simulink model "MMMS_v3"  (R2024b)
settings: Solver=VariableStepAuto  StartTime=0.0  StopTime=60  FixedStep=0.001  RelTol=1e-3
InitFcn:
  | %rho_0t=[0.29;0.29;0.29]; %m
  | %V_0t=[-0.001;-0.001;0];%[-0.0005;-0.0005;0];
  | %w_t=[0;0;-0.002];
  | 
  | 
  | %rho_0t=[0.3;0.3;0.2]; %m
  | %V_0t=[-0.001;-0.001;0];%[-0.0005;-0.0005;0];
  | %w_t=[0;0;-0.001];
values from neighbouring files (symbols this model uses):
  Dt = 0.1    [main_EKF.m]
  Fake_Manip_grad = -0.2.*eye(7)    [Initiate_FQ.m]
  g_cm = zeros(4,4,n)    [Initiate_KUKA_inv.m]    (also in Main_MMMS.m; test_KUKA_elements.m)
  g_It00 = [eye(3) rho_It;0 0 0 1]    [main_EKF.m]
  iota0 = eye(6,6)    [Initiate_KUKA_inv.m]    (also in Main_MMMS.m; test_KUKA_elements.m)
  K_d = 10*[1.3*eye(3) zeros(3);zeros(3) 0.8*eye(3)]    [Initiate_FQ.m]    (also in Initiate_KUKA_inv.m = 5*[0.7*eye(3) zeros(3);zeros(3) 0.5*eye(3)]; MMMS_Initiate_FQ.m; Main_MMMS.m = 5*[0.7*eye(3) zeros(3);zeros(3) 0.5*eye(3)]; test_KUKA_elements.m = 50*[0.7*eye(3) zeros(3);zeros(3) 0.5*eye(3)])
  K_i = 5*[0.1*eye(3) zeros(3);zeros(3) 0.01*eye(3)]    [Initiate_FQ.m]    (also in Initiate_KUKA_inv.m = 5*[0.01*eye(3) zeros(3);zeros(3) 0.001*eye(3)]; MMMS_Initiate_FQ.m; Main_MMMS.m = 5*[0.01*eye(3) zeros(3);zeros(3) 0.001*eye(3)]; test_KUKA_elements.m = 50*[0.01*eye(3) zeros(3);zeros(3) 0.001*eye(3)])
  K_p = 100*[0.1 0 0 0 0 0;0 0.1 0 0 0 0; 0 0 0.1 0 0 0; 0 0 0 0.01 0 0 ... (first row only)    [Initiate_FQ.m]    (also in Initiate_KUKA_inv.m = 5*[0.1 0 0 0 0 0;0 0.1 0 0 0 0; 0 0 0.1 0 0 0; 0 0 0 0.01 0 ; MMMS_Initiate_FQ.m; Main_MMMS.m = 5*[0.1 0 0 0 0 0;0 0.1 0 0 0 0; 0 0 0.1 0 0 0; 0 0 0 0.01 0 ; test_KUKA_elements.m = 50*[0.1 0 0 0 0 0;0 0.1 0 0 0 0; 0 0 0.1 0 0 0; 0 0 0 0.01 0)
  K_w = 200*eye(7)    [Initiate_FQ.m]    (also in MMMS_Initiate_FQ.m)
  K_wd = 2*eye(7)    [Initiate_FQ.m]    (also in MMMS_Initiate_FQ.m)
  m = randn(s,total_time_steps,6)*chol(R)    [main_EKF.m]
  M0 = M_temp.M0.data(:,:,1)    [Initiate_FQ.m]    (also in MMMS_Initiate_FQ.m; test_KUKA_elements.m)
  m0 = robot.Bodies{1,n+1}.Mass    [Initiate_KUKA_inv.m]    (also in Main_MMMS.m; test_KUKA_elements.m)
  m0_frak = diag_M(1:6,1:6)    [Initiate_KUKA_inv.m]    (also in Main_MMMS.m; make_uncertain.m = diag_M_unc(1:6,1:6); test_KUKA_elements.m)
  M0m = M_temp.M0m.data(:,:,1)    [Initiate_FQ.m]    (also in MMMS_Initiate_FQ.m; test_KUKA_elements.m)
  m_diag = diag_M(7:end,7:end)    [Initiate_KUKA_inv.m]    (also in Main_MMMS.m; make_uncertain.m = diag_M_unc(7:end,7:end); test_KUKA_elements.m)
  M_t = (((Adjoint(g_It))'\M_t_body)/(Adjoint(g_It)))    [Initiate_FQ.m]    (also in Initiate_KUKA_inv.m = [eye(3)*mt zeros(3); zeros(3) eye(3)*80]; MMMS_Initiate_FQ.m; Main_MMMS.m = [eye(3)*mt zeros(3); zeros(3) eye(3)*80]; test_KUKA_elements.m = [eye(3)*mt zeros(3); zeros(3) eye(3)*80])
  M_t_body = [eye(3)*mt zeros(3); zeros(3) eye(3)*0.416667]    [Initiate_FQ.m]    (also in MMMS_Initiate_FQ.m)
  mm = zeros(1,n)    [Initiate_KUKA_inv.m]    (also in Main_MMMS.m; test_KUKA_elements.m)
  mu = P0    [Initiate_FQ.m]    (also in Initiate_KUKA_inv.m = zeros(6,1); MMMS_Initiate_FQ.m; Main_MMMS.m = zeros(6,1); make_uncertain.m = P0_unc)
  mu_t = inv((Adjoint(g_It))')*M_t_body*[V_It;w_t]    [Initiate_FQ.m]    (also in Initiate_KUKA_inv.m = M_t*[V_0t;w_t]; MMMS_Initiate_FQ.m; Main_MMMS.m = M_t*[V_0t;w_t]; make_uncertain.m = inv((Adjoint(g_It))')*M_t_body_unc*[V_It;w_t])
  noise_st = 0.000005    (= 5e-06)    [main_EKF.m]
  q_dot_m = [0;0;0;0;0;0;0]    [Initiate_FQ.m]    (also in Initiate_KUKA_inv.m; MMMS_Initiate_FQ.m; Main_MMMS.m; test_KUKA_elements.m = [0])
  q_m = [0.2;1.2;0.3;2.5;0.5;1.5;0.6]    [Initiate_FQ.m]    (also in Initiate_KUKA_inv.m = [0;0;0;0;0;0;0]; MMMS_Initiate_FQ.m = [0.2;0.2;0.3;0.5;0.5;0.5;0.6]; Main_MMMS.m = [0;0;0;0;0;0;0]; test_KUKA_elements.m = [0.2;1.2;0.3;1.8;0.5;1.3;0.6])
  rho_It = [0;0;1.7]    [Initiate_FQ.m]    (also in MMMS_Initiate_FQ.m)
  s = RandStream.create('mrg32k3a','NumStreams',1)    [main_EKF.m]
  sc_size = 1    [Initiate_KUKA_inv.m]    (also in Main_MMMS.m; test_KUKA_elements.m)
  V_It = [0.0005;0.0005;0]    [Initiate_FQ.m]    (also in MMMS_Initiate_FQ.m = [0.001;0.001;0])
  Xi_m_matrix = zeros(6*n,n)    [Initiate_KUKA_inv.m]    (also in Main_MMMS.m)
undefined symbols (not defined in the file or in its folder): g_cm0, I0, Im, Mm, X, Xi_m, Y, Z
libraries: nesl_utility x314, sm_lib x231, robotcorelib x30, simulink x12
(part 2 of 13)

== system MMMS_v3/Feedback Transformation1 ==
  note: Feedback Transformation
  g_I0 : Inport
  q_m : Inport  Port=2
  U_c2 : Inport  Port=3
  f_N : Inport  Port=4
  CBF_m : Inport  Port=5
  Add1 : Sum  Inputs=+++++++
  Bus Selector1 : BusSelector  OutputSignals=signal2
  Constant1 : Constant  Value=mu
  Constant4 : Constant  Value=mu_t
  Gain10 : Gain
  Gain5 : Gain  Gain=0
  Gain7 : Gain  Gain=0
  Gain8 : Gain
  Gain9 : Gain  Gain=0
  Inverse Dynamics1 : Subsystem
  Matrix Multiply{1..3,8} (4 alike) : Product  Multiplication=Matrix(*)
  f_m : Outport
  tag scope: fm2=global
  wires:
  q_m/1 -> Inverse Dynamics1/2("q_m "), Bus Selector1/1
  g_I0/1 -> Inverse Dynamics1/1(g_I0)
  Gain8/1 -> Add1/5
  Inverse Dynamics1/3(F_t) -> Matrix Multiply8/1
  Inverse Dynamics1/4(F_m) -> Matrix Multiply1/1
  Gain9/1 -> Add1/4
  Constant4/1 -> Matrix Multiply8/2  "mu_t"
  Add1/1 -> [fm2], f_m/1  "f_m"
  Bus Selector1/1 -> Matrix Multiply1/2  "<signal2>"
  f_N/1 -> Gain10/1
  Gain5/1 -> Add1/1
  Matrix Multiply3/1 -> Gain9/1
  Matrix Multiply8/1 -> Gain8/1
  Inverse Dynamics1/5(N) -> Gain5/1
  U_c2/1 -> Matrix Multiply2/2
  Constant1/1 -> Matrix Multiply3/2  "mu"
  Inverse Dynamics1/1(F_U) -> Matrix Multiply2/1
  Gain10/1 -> Add1/6
  Matrix Multiply1/1 -> Gain7/1
  Gain7/1 -> Add1/2
  Inverse Dynamics1/2(F_mu) -> Matrix Multiply3/1
  CBF_m/1 -> Add1/7
  Matrix Multiply2/1 -> Add1/3  "f_m"

== system MMMS_v3/Feedback Transformation2 ==
  note: Feedback Transformation
  g_I0 : Inport
  q_m : Inport  Port=2
  U_c2 : Inport  Port=3
  f_N : Inport  Port=4
  Add1 : Sum  Inputs=++++++
  Bus Selector1 : BusSelector  OutputSignals=signal2
  Constant1 : Constant  Value=mu
  Constant4 : Constant  Value=mu_t
  Gain10 : Gain
  Gain5 : Gain  Gain=0
  Gain7 : Gain  Gain=0
  Gain8 : Gain
  Gain9 : Gain  Gain=0
  Inverse Dynamics1 : Subsystem
  Matrix Multiply{1..3,8} (4 alike) : Product  Multiplication=Matrix(*)
  f_m : Outport
  tag scope: fm3=global
  wires:
  Inverse Dynamics1/2(F_mu) -> Matrix Multiply3/1
  Gain7/1 -> Add1/2
  Matrix Multiply1/1 -> Gain7/1
  Gain10/1 -> Add1/6
  Inverse Dynamics1/1(F_U) -> Matrix Multiply2/1
  Constant1/1 -> Matrix Multiply3/2  "mu"
  U_c2/1 -> Matrix Multiply2/2
  Inverse Dynamics1/5(N) -> Gain5/1
  Matrix Multiply8/1 -> Gain8/1
  Matrix Multiply3/1 -> Gain9/1
  Gain5/1 -> Add1/1
  f_N/1 -> Gain10/1
  Matrix Multiply2/1 -> Add1/3  "f_m"
  Bus Selector1/1 -> Matrix Multiply1/2  "<signal2>"
  Add1/1 -> [fm3], f_m/1  "f_m"
  Constant4/1 -> Matrix Multiply8/2  "mu_t"
  Gain9/1 -> Add1/4
  Inverse Dynamics1/4(F_m) -> Matrix Multiply1/1
  Inverse Dynamics1/3(F_t) -> Matrix Multiply8/1
  Gain8/1 -> Add1/5
  g_I0/1 -> Inverse Dynamics1/1(g_I0)
  q_m/1 -> Bus Selector1/1, Inverse Dynamics1/2("q_m ")

== system MMMS_v3/Inverse Dynamics ==
  note: f_m
  g_I0 : Inport
  "q_m " : Inport  Port=2
  A_dot : MATLAB Function  TreatAsAtomicUnit=on
  Bus Selector : BusSelector  OutputSignals=M0,Mm
  Bus Selector2 : BusSelector  OutputSignals=signal1,signal2
  C_hat : Subsystem  Commented=on
  C_hat1 : Subsystem
  Inverse Dynamics : Subsystem
  M0_dot : MATLAB Function  TreatAsAtomicUnit=on
  N_hat : Subsystem  Commented=on
  N_hat1 : Subsystem
  Scope : Scope
  F_U : Outport
  F_mu : Outport  Port=2
  F_t : Outport  Port=3
  F_m : Outport  Port=4
  N : Outport  Port=5
  wires:
  [P] -> N_hat1/5(P)
  [Mass_Matrix] -> Bus Selector/1
  Bus Selector/1 -> N_hat1/6(M0), Inverse Dynamics/2(<M0>)  "<M0>"
  g_I0/1 -> N_hat1/1(g_I0), Inverse Dynamics/1(g_I0)
  Inverse Dynamics/1(F_U) -> F_U/1
  Inverse Dynamics/2(F_mu) -> F_mu/1
  Inverse Dynamics/3(F_t) -> F_t/1
  Inverse Dynamics/4(F_m) -> F_m/1
  Bus Selector/2 -> Inverse Dynamics/3(Mm)  "<Mm>"
  Bus Selector2/1 -> N_hat1/2(q_m), C_hat1/1(q_m)  "<signal1>"
  Bus Selector2/2 -> A_dot/2(q_m_dot), M0_dot/2(q_m_dot), N_hat1/3(q_dot_m), C_hat1/2(q_dot_m)  "<signal2>"
  C_hat1/1(M0_partial) -> M0_dot/1(M0_partial)
  C_hat1/2(Out1) -> A_dot/1(A_partial)
  C_hat1/3(C_hat1) -> Inverse Dynamics/6(C_hat)
  M0_dot/1(M0_dot) -> Inverse Dynamics/4(M0_dot)
  A_dot/1(A_dot) -> Inverse Dynamics/5(A_dot)
  "q_m "/1 -> Bus Selector2/1
  [A_connection] -> N_hat1/4(A)
  N_hat1/1(N_hat1) -> N/1, Scope/1

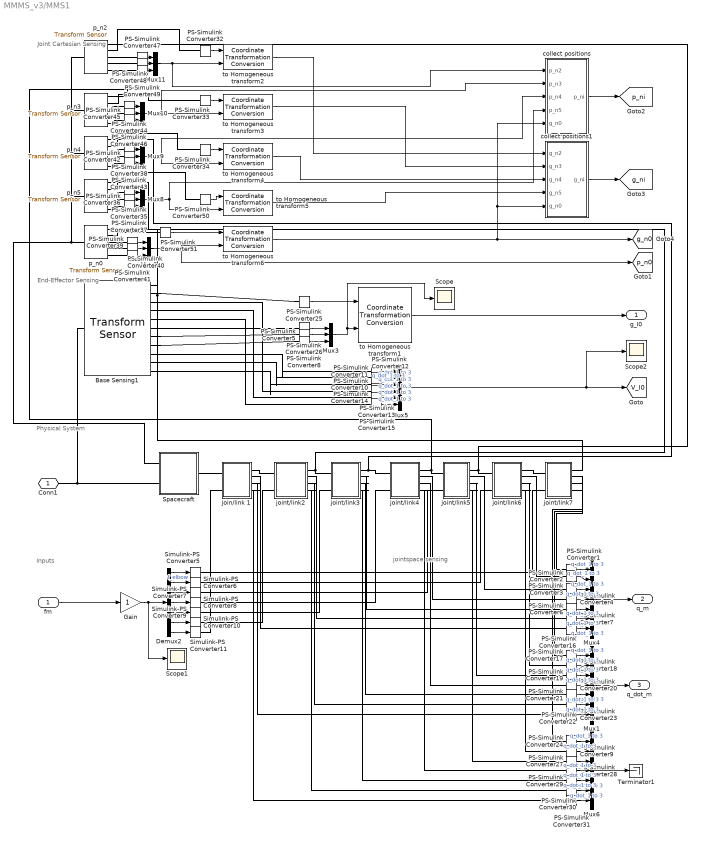
== system MMMS_v3/MMS1 ==
  note: Physical System
  note: jointspace sensing
  note: Inputs
  note: End-Effector Sensing
  note: Joint Cartesian Sensing
  fm : Inport
  Base Sensing1 : sm_lib/Frames and Transforms/Transform Sensor  MeasurementFrame=NonRotatingBase  RotationSequence=XYZ  SenseAngle=off  SenseAxis=off  SenseQ=off  SenseR=on  SenseRotationSequence=off  SenseOmegaX=on  SenseOmegaY=on  SenseOmegaZ=on  SenseOmega=off  SenseQDot=off  SenseRDot=off  SenseRotationSequenceDot=off  SenseAlphaX=off  SenseAlphaY=off  SenseAlphaZ=off  SenseAlpha=off  SenseQDDot=off  SenseRDDot=off  SenseX=on  SenseY=on  SenseZ=on  SenseXYZ=off  SenseRad=off  SenseAzim=off  SenseDist=off  SenseInc=off  SenseXDot=on  SenseYDot=on  SenseZDot=on  SenseXYZDot=off  SenseRadDot=off  SenseAzimDot=off  SenseDistDot=off  SenseIncDot=off  SenseXDDot=off  SenseYDDot=off  SenseZDDot=off  SenseXYZDDot=off  SenseRadDDot=off  SenseAzimDDot=off  SenseDistDDot=off  SenseIncDDot=off
  Demux2 : Demux  Outputs=7
  Gain : Gain
  Mux1 : Mux  Inputs=7
  Mux{2..3,8..11} (6 alike) : Mux  Inputs=3
  Mux4 : Mux  Inputs=7
  Mux5 : Mux  Inputs=6
  Mux6 : Mux  Inputs=7
  PS-Simulink Converter{1..51} (51 alike) : nesl_utility/PS-Simulink Converter  PhysicalDomain=network_engine_domain  SubClassName=ps_output  LeftPortType=input  RightPortType=output  PseudoPeriodic=off  Frequencies=[]  VectorFormat=1-D array  Unit=inherit  AffineConversion=off
  Scope : Scope
  Scope1 : Scope
  Scope2 : Scope
  Simulink-PS Converter{5..11} (7 alike) : nesl_utility/Simulink-PS Converter  PhysicalDomain=network_engine_domain  SubClassName=ps_input  LeftPortType=input  RightPortType=output  PseudoPeriodic=off  Frequencies=[]  NoiseDistribution=none  NoiseParameters=[]  Unit=1  AffineConversion=off  FilteringAndDerivatives=provide  SimscapeFilterOrder=1  InputFilterTimeConstant=0.001  UdotUserProvided=0
  Spacecraft : Subsystem
  Terminator1 : Terminator
  collect positions : MATLAB Function  TreatAsAtomicUnit=on
  collect positions1 : MATLAB Function  TreatAsAtomicUnit=on
  join/link 1 : Subsystem
  joint/link2 : Subsystem
  joint/link3 : Subsystem
  joint/link4 : Subsystem
  joint/link5 : Subsystem
  joint/link6 : Subsystem
  joint/link7 : Subsystem
  p_n{0,2..5} (5 alike) : sm_lib/Frames and Transforms/Transform Sensor  MeasurementFrame=Base  RotationSequence=XYZ  SenseAngle=off  SenseAxis=off  SenseQ=off  SenseR=on  SenseRotationSequence=off  SenseOmegaX=off  SenseOmegaY=off  SenseOmegaZ=off  SenseOmega=off  SenseQDot=off  SenseRDot=off  SenseRotationSequenceDot=off  SenseAlphaX=off  SenseAlphaY=off  SenseAlphaZ=off  SenseAlpha=off  SenseQDDot=off  SenseRDDot=off  SenseX=on  SenseY=on  SenseZ=on  SenseXYZ=off  SenseRad=off  SenseAzim=off  SenseDist=off  SenseInc=off  SenseXDot=off  SenseYDot=off  SenseZDot=off  SenseXYZDot=off  SenseRadDot=off  SenseAzimDot=off  SenseDistDot=off  SenseIncDot=off  SenseXDDot=off  SenseYDDot=off  SenseZDDot=off  SenseXYZDDot=off  SenseRadDDot=off  SenseAzimDDot=off  SenseDistDDot=off  SenseIncDDot=off
  to Homogeneous transform{1..6} (6 alike) : robotcorelib/Coordinate Transformation Conversion  InputRepresentation=Rotation Matrix  InputEulerSequence=ZYX  ShowTrVecInputPort=on  OutputRepresentation=Homogeneous Transformation  OutputEulerSequence=ZYX  ShowTrVecOutputPort=on  SimulateUsing=Code generation
  Conn1 : PMIOPort  Side=Left
  g_I0 : Outport
  q_m : Outport  Port=2
  q_dot_m : Outport  Port=3
  tag scope: V_I0=global, g_n0=global, g_ni=global, p_n0=global, p_ni=global
  wires:
  Demux2/1 -> Simulink-PS Converter5/1
  Demux2/3 -> Simulink-PS Converter7/1
  PS-Simulink Converter15/1 -> Mux5/6  "q_dot_1 to 3"
  PS-Simulink Converter10/1 -> Mux5/3  "q_dot_1 to 3"
  fm/1 -> Gain/1
  PS-Simulink Converter25/1 -> to Homogeneous transform1/1
  Gain/1 -> Scope1/1, Demux2/1
  PS-Simulink Converter8/1 -> Mux3/3
  Mux3/1 -> Scope/1, to Homogeneous transform1/2
  PS-Simulink Converter12/1 -> Mux5/2  "q_dot_1 to 3"
  to Homogeneous transform1/1 -> g_I0/1
  PS-Simulink Converter13/1 -> Mux5/4  "q_dot_1 to 3"
  PS-Simulink Converter26/1 -> Mux3/1
  Demux2/7 -> Simulink-PS Converter11/1
  PS-Simulink Converter14/1 -> Mux5/5  "q_dot_1 to 3"
  Demux2/4 -> Simulink-PS Converter8/1
  PS-Simulink Converter11/1 -> Mux5/1  "q_dot_1 to 3"
  PS-Simulink Converter5/1 -> Mux3/2
  Demux2/6 -> Simulink-PS Converter10/1
  Demux2/2 -> Simulink-PS Converter6/1  "f_elbow"
  Demux2/5 -> Simulink-PS Converter9/1
  PS-Simulink Converter27/1 -> Mux6/3  "q_dot_1 to 3"
  PS-Simulink Converter1/1 -> Mux4/1  "q_dot_1 to 3"
  PS-Simulink Converter6/1 -> Mux4/5  "q_dot_1 to 3"
  PS-Simulink Converter30/1 -> Mux6/6  "q_dot_1 to 3"
  PS-Simulink Converter3/1 -> Mux4/3  "q_dot_1 to 3"
  PS-Simulink Converter18/1 -> Mux1/2  "q_dot_1 to 3"
  PS-Simulink Converter31/1 -> Mux6/7  "q_dot_1 to 3"
  PS-Simulink Converter9/1 -> Mux6/2  "q_dot_1 to 3"
  PS-Simulink Converter7/1 -> Mux4/6  "q_dot_1 to 3"
  PS-Simulink Converter2/1 -> Mux4/2  "q_dot_1 to 3"
  PS-Simulink Converter4/1 -> Mux4/4  "q_dot_1 to 3"
  PS-Simulink Converter21/1 -> Mux1/5  "q_dot_1 to 3"
  PS-Simulink Converter23/1 -> Mux1/7  "q_dot_1 to 3"
  PS-Simulink Converter16/1 -> Mux4/7  "q_dot_1 to 3"
  PS-Simulink Converter28/1 -> Mux6/4  "q_dot_1 to 3"
  Mux4/1 -> q_m/1
  Mux1/1 -> q_dot_m/1
  PS-Simulink Converter24/1 -> Mux6/1  "q_dot_1 to 3"
  Mux6/1 -> Terminator1/1
  PS-Simulink Converter20/1 -> Mux1/4  "q_dot_1 to 3"
  PS-Simulink Converter29/1 -> Mux6/5  "q_dot_1 to 3"
  PS-Simulink Converter22/1 -> Mux1/6  "q_dot_1 to 3"
  PS-Simulink Converter17/1 -> Mux1/1  "q_dot_1 to 3"
  PS-Simulink Converter19/1 -> Mux1/3  "q_dot_1 to 3"
  Mux5/1 -> [V_I0], Scope2/1
  Mux2/1 -> to Homogeneous transform6/2, [p_n0]
  PS-Simulink Converter39/1 -> Mux2/1
  PS-Simulink Converter40/1 -> Mux2/2
  PS-Simulink Converter41/1 -> Mux2/3
  PS-Simulink Converter36/1 -> Mux8/2
  PS-Simulink Converter35/1 -> Mux8/1
  PS-Simulink Converter37/1 -> Mux8/3
  PS-Simulink Converter42/1 -> Mux9/2
  PS-Simulink Converter38/1 -> Mux9/1
  PS-Simulink Converter43/1 -> Mux9/3
  PS-Simulink Converter45/1 -> Mux10/2
  PS-Simulink Converter44/1 -> Mux10/1
  PS-Simulink Converter46/1 -> Mux10/3
  Mux11/1 -> to Homogeneous transform2/2, collect positions/1(p_n2)
  PS-Simulink Converter48/1 -> Mux11/2
  PS-Simulink Converter47/1 -> Mux11/1
  PS-Simulink Converter49/1 -> Mux11/3
  collect positions/1(p_ni) -> [p_ni]
  PS-Simulink Converter32/1 -> to Homogeneous transform2/1
  PS-Simulink Converter33/1 -> to Homogeneous transform3/1
  Mux10/1 -> to Homogeneous transform3/2, collect positions/2(p_n3)
  Mux9/1 -> to Homogeneous transform4/2, collect positions/3(p_n4)
  PS-Simulink Converter34/1 -> to Homogeneous transform4/1
  PS-Simulink Converter50/1 -> to Homogeneous transform5/1
  Mux8/1 -> to Homogeneous transform5/2, collect positions/4(p_n5)
  collect positions1/1(g_ni) -> [g_ni]
  PS-Simulink Converter51/1 -> to Homogeneous transform6/1
  to Homogeneous transform6/1 -> collect positions/5(g_n0), collect positions1/5(g_n0), [g_n0]
  to Homogeneous transform2/1 -> collect positions1/1(g_n2)
  to Homogeneous transform3/1 -> collect positions1/2(g_n3)
  to Homogeneous transform4/1 -> collect positions1/3(g_n4)
  to Homogeneous transform5/1 -> collect positions1/4(g_n5)
  connections:
  Spacecraft/LConn2 -- Conn1/RConn1 -- Base Sensing1/LConn1
  p_n0/RConn1 -- joint/link7/RConn1 -- Base Sensing1/RConn1
  joint/link4/LConn1 -- p_n4/RConn1 -- joint/link3/RConn1
  Base Sensing1/RConn10 -- PS-Simulink Converter12/LConn1
  Simulink-PS Converter9/RConn1 -- joint/link3/LConn2
  Simulink-PS Converter8/RConn1 -- joint/link4/LConn2
  Base Sensing1/RConn2 -- PS-Simulink Converter25/LConn1
  joint/link5/LConn1 -- joint/link4/RConn1 -- p_n3/RConn1
  Base Sensing1/RConn5 -- PS-Simulink Converter15/LConn1
  Base Sensing1/RConn7 -- PS-Simulink Converter5/LConn1
  joint/link6/LConn1 -- joint/link5/RConn1 -- p_n2/RConn1
  Base Sensing1/RConn11 -- PS-Simulink Converter10/LConn1
  Base Sensing1/RConn3 -- PS-Simulink Converter13/LConn1
  Simulink-PS Converter5/RConn1 -- joint/link7/LConn2
  Base Sensing1/RConn4 -- PS-Simulink Converter14/LConn1
  Base Sensing1/RConn9 -- PS-Simulink Converter11/LConn1
  Base Sensing1/RConn8 -- PS-Simulink Converter8/LConn1
  Base Sensing1/RConn6 -- PS-Simulink Converter26/LConn1
  Simulink-PS Converter7/RConn1 -- joint/link5/LConn2
  joint/link6/RConn3 -- PS-Simulink Converter18/LConn1
  joint/link6/RConn4 -- PS-Simulink Converter9/LConn1
  joint/link5/RConn2 -- PS-Simulink Converter3/LConn1
  joint/link5/RConn3 -- PS-Simulink Converter19/LConn1
  joint/link5/RConn4 -- PS-Simulink Converter27/LConn1
  joint/link4/RConn2 -- PS-Simulink Converter4/LConn1
  joint/link4/RConn3 -- PS-Simulink Converter20/LConn1
  joint/link4/RConn4 -- PS-Simulink Converter28/LConn1
  joint/link3/RConn2 -- PS-Simulink Converter6/LConn1
  joint/link3/RConn3 -- PS-Simulink Converter21/LConn1
  joint/link3/RConn4 -- PS-Simulink Converter29/LConn1
  joint/link6/RConn1 -- joint/link7/LConn1
  joint/link6/RConn2 -- PS-Simulink Converter2/LConn1
  joint/link6/LConn2 -- Simulink-PS Converter6/RConn1
  joint/link7/RConn2 -- PS-Simulink Converter1/LConn1
  joint/link7/RConn3 -- PS-Simulink Converter17/LConn1
  joint/link7/RConn4 -- PS-Simulink Converter24/LConn1
  join/link 1/LConn2 -- Simulink-PS Converter11/RConn1
  join/link 1/LConn1 -- Spacecraft/RConn1
  join/link 1/RConn1 -- joint/link2/LConn1
  Simulink-PS Converter10/RConn1 -- joint/link2/LConn2
  joint/link3/LConn1 -- p_n5/RConn1 -- joint/link2/RConn1
  join/link 1/RConn2 -- PS-Simulink Converter16/LConn1
  PS-Simulink Converter7/LConn1 -- joint/link2/RConn2
  joint/link2/RConn4 -- PS-Simulink Converter30/LConn1
  join/link 1/RConn4 -- PS-Simulink Converter31/LConn1
  joint/link2/RConn3 -- PS-Simulink Converter22/LConn1
  join/link 1/RConn3 -- PS-Simulink Converter23/LConn1
  PS-Simulink Converter41/LConn1 -- p_n0/RConn5
  p_n0/RConn4 -- PS-Simulink Converter40/LConn1
  Spacecraft/LConn1 -- p_n2/LConn1 -- p_n3/LConn1 -- p_n4/LConn1 -- p_n5/LConn1 -- p_n0/LConn1
  p_n0/RConn3 -- PS-Simulink Converter39/LConn1
  PS-Simulink Converter37/LConn1 -- p_n5/RConn5
  p_n5/RConn3 -- PS-Simulink Converter35/LConn1
  p_n5/RConn4 -- PS-Simulink Converter36/LConn1
  PS-Simulink Converter43/LConn1 -- p_n4/RConn5
  p_n4/RConn3 -- PS-Simulink Converter38/LConn1
  p_n4/RConn4 -- PS-Simulink Converter42/LConn1
  PS-Simulink Converter46/LConn1 -- p_n3/RConn5
  p_n3/RConn3 -- PS-Simulink Converter44/LConn1
  p_n3/RConn4 -- PS-Simulink Converter45/LConn1
  PS-Simulink Converter49/LConn1 -- p_n2/RConn5
  p_n2/RConn3 -- PS-Simulink Converter47/LConn1
  p_n2/RConn4 -- PS-Simulink Converter48/LConn1
  PS-Simulink Converter32/LConn1 -- p_n2/RConn2
  p_n3/RConn2 -- PS-Simulink Converter33/LConn1
  p_n4/RConn2 -- PS-Simulink Converter34/LConn1
  p_n5/RConn2 -- PS-Simulink Converter50/LConn1
  p_n0/RConn2 -- PS-Simulink Converter51/LConn1

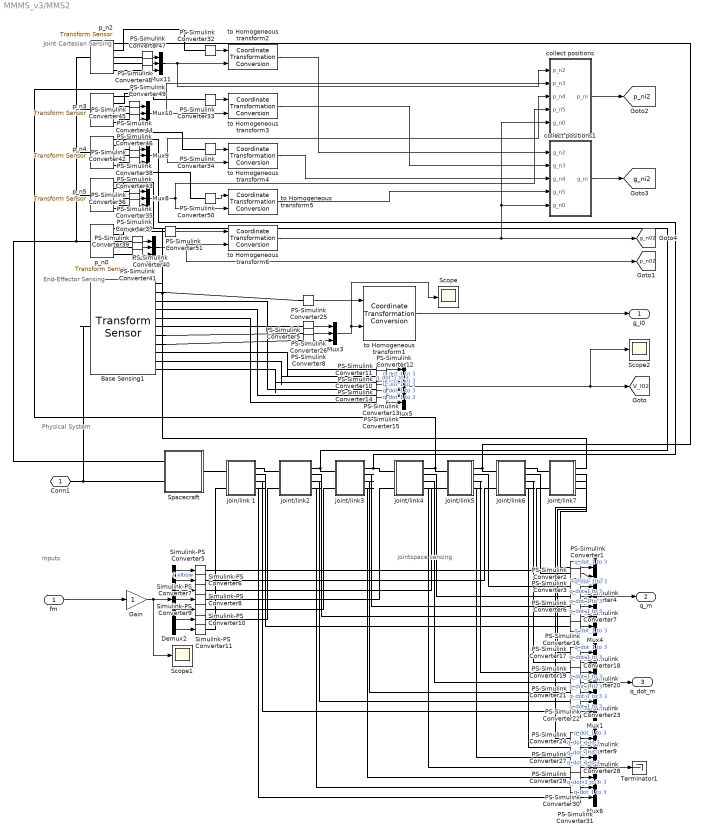
== system MMMS_v3/MMS2 ==
  note: Joint Cartesian Sensing
  note: End-Effector Sensing
  note: Inputs
  note: jointspace sensing
  note: Physical System
  fm : Inport
  Base Sensing1 : sm_lib/Frames and Transforms/Transform Sensor  MeasurementFrame=NonRotatingBase  RotationSequence=XYZ  SenseAngle=off  SenseAxis=off  SenseQ=off  SenseR=on  SenseRotationSequence=off  SenseOmegaX=on  SenseOmegaY=on  SenseOmegaZ=on  SenseOmega=off  SenseQDot=off  SenseRDot=off  SenseRotationSequenceDot=off  SenseAlphaX=off  SenseAlphaY=off  SenseAlphaZ=off  SenseAlpha=off  SenseQDDot=off  SenseRDDot=off  SenseX=on  SenseY=on  SenseZ=on  SenseXYZ=off  SenseRad=off  SenseAzim=off  SenseDist=off  SenseInc=off  SenseXDot=on  SenseYDot=on  SenseZDot=on  SenseXYZDot=off  SenseRadDot=off  SenseAzimDot=off  SenseDistDot=off  SenseIncDot=off  SenseXDDot=off  SenseYDDot=off  SenseZDDot=off  SenseXYZDDot=off  SenseRadDDot=off  SenseAzimDDot=off  SenseDistDDot=off  SenseIncDDot=off
  Demux2 : Demux  Outputs=7
  Gain : Gain
  Mux1 : Mux  Inputs=7
  Mux{2..3,8..11} (6 alike) : Mux  Inputs=3
  Mux4 : Mux  Inputs=7
  Mux5 : Mux  Inputs=6
  Mux6 : Mux  Inputs=7
  PS-Simulink Converter{1..51} (51 alike) : nesl_utility/PS-Simulink Converter  PhysicalDomain=network_engine_domain  SubClassName=ps_output  LeftPortType=input  RightPortType=output  PseudoPeriodic=off  Frequencies=[]  VectorFormat=1-D array  Unit=inherit  AffineConversion=off
  Scope : Scope
  Scope1 : Scope
  Scope2 : Scope
  Simulink-PS Converter{5..11} (7 alike) : nesl_utility/Simulink-PS Converter  PhysicalDomain=network_engine_domain  SubClassName=ps_input  LeftPortType=input  RightPortType=output  PseudoPeriodic=off  Frequencies=[]  NoiseDistribution=none  NoiseParameters=[]  Unit=1  AffineConversion=off  FilteringAndDerivatives=provide  SimscapeFilterOrder=1  InputFilterTimeConstant=0.001  UdotUserProvided=0
  Spacecraft : Subsystem
  Terminator1 : Terminator
  collect positions : MATLAB Function  TreatAsAtomicUnit=on
  collect positions1 : MATLAB Function  TreatAsAtomicUnit=on
  join/link 1 : Subsystem
  joint/link2 : Subsystem
  joint/link3 : Subsystem
  joint/link4 : Subsystem
  joint/link5 : Subsystem
  joint/link6 : Subsystem
  joint/link7 : Subsystem
  p_n{0,2..5} (5 alike) : sm_lib/Frames and Transforms/Transform Sensor  MeasurementFrame=Base  RotationSequence=XYZ  SenseAngle=off  SenseAxis=off  SenseQ=off  SenseR=on  SenseRotationSequence=off  SenseOmegaX=off  SenseOmegaY=off  SenseOmegaZ=off  SenseOmega=off  SenseQDot=off  SenseRDot=off  SenseRotationSequenceDot=off  SenseAlphaX=off  SenseAlphaY=off  SenseAlphaZ=off  SenseAlpha=off  SenseQDDot=off  SenseRDDot=off  SenseX=on  SenseY=on  SenseZ=on  SenseXYZ=off  SenseRad=off  SenseAzim=off  SenseDist=off  SenseInc=off  SenseXDot=off  SenseYDot=off  SenseZDot=off  SenseXYZDot=off  SenseRadDot=off  SenseAzimDot=off  SenseDistDot=off  SenseIncDot=off  SenseXDDot=off  SenseYDDot=off  SenseZDDot=off  SenseXYZDDot=off  SenseRadDDot=off  SenseAzimDDot=off  SenseDistDDot=off  SenseIncDDot=off
  to Homogeneous transform{1..6} (6 alike) : robotcorelib/Coordinate Transformation Conversion  InputRepresentation=Rotation Matrix  InputEulerSequence=ZYX  ShowTrVecInputPort=on  OutputRepresentation=Homogeneous Transformation  OutputEulerSequence=ZYX  ShowTrVecOutputPort=on  SimulateUsing=Code generation
  Conn1 : PMIOPort  Side=Left
  g_I0 : Outport
  q_m : Outport  Port=2
  q_dot_m : Outport  Port=3
  tag scope: V_I02=global, g_n02=global, g_ni2=global, p_n02=global, p_ni2=global
  wires:
  to Homogeneous transform5/1 -> collect positions1/4(g_n5)
  to Homogeneous transform4/1 -> collect positions1/3(g_n4)
  to Homogeneous transform3/1 -> collect positions1/2(g_n3)
  to Homogeneous transform2/1 -> collect positions1/1(g_n2)
  to Homogeneous transform6/1 -> [g_n02], collect positions1/5(g_n0), collect positions/5(g_n0)
  PS-Simulink Converter51/1 -> to Homogeneous transform6/1
  collect positions1/1(g_ni) -> [g_ni2]
  Mux8/1 -> collect positions/4(p_n5), to Homogeneous transform5/2
  PS-Simulink Converter50/1 -> to Homogeneous transform5/1
  PS-Simulink Converter34/1 -> to Homogeneous transform4/1
  Mux9/1 -> collect positions/3(p_n4), to Homogeneous transform4/2
  Mux10/1 -> collect positions/2(p_n3), to Homogeneous transform3/2
  PS-Simulink Converter33/1 -> to Homogeneous transform3/1
  PS-Simulink Converter32/1 -> to Homogeneous transform2/1
  collect positions/1(p_ni) -> [p_ni2]
  PS-Simulink Converter49/1 -> Mux11/3
  PS-Simulink Converter47/1 -> Mux11/1
  PS-Simulink Converter48/1 -> Mux11/2
  Mux11/1 -> collect positions/1(p_n2), to Homogeneous transform2/2
  PS-Simulink Converter46/1 -> Mux10/3
  PS-Simulink Converter44/1 -> Mux10/1
  PS-Simulink Converter45/1 -> Mux10/2
  PS-Simulink Converter43/1 -> Mux9/3
  PS-Simulink Converter38/1 -> Mux9/1
  PS-Simulink Converter42/1 -> Mux9/2
  PS-Simulink Converter37/1 -> Mux8/3
  PS-Simulink Converter35/1 -> Mux8/1
  PS-Simulink Converter36/1 -> Mux8/2
  PS-Simulink Converter41/1 -> Mux2/3
  PS-Simulink Converter40/1 -> Mux2/2
  PS-Simulink Converter39/1 -> Mux2/1
  Mux2/1 -> [p_n02], to Homogeneous transform6/2
  Mux5/1 -> Scope2/1, [V_I02]
  PS-Simulink Converter19/1 -> Mux1/3  "q_dot_1 to 3"
  PS-Simulink Converter17/1 -> Mux1/1  "q_dot_1 to 3"
  PS-Simulink Converter22/1 -> Mux1/6  "q_dot_1 to 3"
  PS-Simulink Converter29/1 -> Mux6/5  "q_dot_1 to 3"
  PS-Simulink Converter20/1 -> Mux1/4  "q_dot_1 to 3"
  Mux6/1 -> Terminator1/1
  PS-Simulink Converter24/1 -> Mux6/1  "q_dot_1 to 3"
  Mux1/1 -> q_dot_m/1
  Mux4/1 -> q_m/1
  PS-Simulink Converter28/1 -> Mux6/4  "q_dot_1 to 3"
  PS-Simulink Converter16/1 -> Mux4/7  "q_dot_1 to 3"
  PS-Simulink Converter23/1 -> Mux1/7  "q_dot_1 to 3"
  PS-Simulink Converter21/1 -> Mux1/5  "q_dot_1 to 3"
  PS-Simulink Converter4/1 -> Mux4/4  "q_dot_1 to 3"
  PS-Simulink Converter2/1 -> Mux4/2  "q_dot_1 to 3"
  PS-Simulink Converter7/1 -> Mux4/6  "q_dot_1 to 3"
  PS-Simulink Converter9/1 -> Mux6/2  "q_dot_1 to 3"
  PS-Simulink Converter31/1 -> Mux6/7  "q_dot_1 to 3"
  PS-Simulink Converter18/1 -> Mux1/2  "q_dot_1 to 3"
  PS-Simulink Converter3/1 -> Mux4/3  "q_dot_1 to 3"
  PS-Simulink Converter30/1 -> Mux6/6  "q_dot_1 to 3"
  PS-Simulink Converter6/1 -> Mux4/5  "q_dot_1 to 3"
  PS-Simulink Converter1/1 -> Mux4/1  "q_dot_1 to 3"
  PS-Simulink Converter27/1 -> Mux6/3  "q_dot_1 to 3"
  Demux2/5 -> Simulink-PS Converter9/1
  Demux2/2 -> Simulink-PS Converter6/1  "f_elbow"
  Demux2/6 -> Simulink-PS Converter10/1
  PS-Simulink Converter5/1 -> Mux3/2
  PS-Simulink Converter11/1 -> Mux5/1  "q_dot_1 to 3"
  Demux2/4 -> Simulink-PS Converter8/1
  PS-Simulink Converter14/1 -> Mux5/5  "q_dot_1 to 3"
  Demux2/7 -> Simulink-PS Converter11/1
  PS-Simulink Converter26/1 -> Mux3/1
  PS-Simulink Converter13/1 -> Mux5/4  "q_dot_1 to 3"
  to Homogeneous transform1/1 -> g_I0/1
  PS-Simulink Converter12/1 -> Mux5/2  "q_dot_1 to 3"
  Mux3/1 -> to Homogeneous transform1/2, Scope/1
  PS-Simulink Converter8/1 -> Mux3/3
  Gain/1 -> Demux2/1, Scope1/1
  PS-Simulink Converter25/1 -> to Homogeneous transform1/1
  fm/1 -> Gain/1
  PS-Simulink Converter10/1 -> Mux5/3  "q_dot_1 to 3"
  PS-Simulink Converter15/1 -> Mux5/6  "q_dot_1 to 3"
  Demux2/3 -> Simulink-PS Converter7/1
  Demux2/1 -> Simulink-PS Converter5/1
  connections:
  p_n0/RConn2 -- PS-Simulink Converter51/LConn1
  p_n5/RConn2 -- PS-Simulink Converter50/LConn1
  p_n4/RConn2 -- PS-Simulink Converter34/LConn1
  p_n3/RConn2 -- PS-Simulink Converter33/LConn1
  PS-Simulink Converter32/LConn1 -- p_n2/RConn2
  p_n2/RConn4 -- PS-Simulink Converter48/LConn1
  p_n2/RConn3 -- PS-Simulink Converter47/LConn1
  PS-Simulink Converter49/LConn1 -- p_n2/RConn5
  p_n3/RConn4 -- PS-Simulink Converter45/LConn1
  p_n3/RConn3 -- PS-Simulink Converter44/LConn1
  PS-Simulink Converter46/LConn1 -- p_n3/RConn5
  p_n4/RConn4 -- PS-Simulink Converter42/LConn1
  p_n4/RConn3 -- PS-Simulink Converter38/LConn1
  PS-Simulink Converter43/LConn1 -- p_n4/RConn5
  p_n5/RConn4 -- PS-Simulink Converter36/LConn1
  p_n5/RConn3 -- PS-Simulink Converter35/LConn1
  PS-Simulink Converter37/LConn1 -- p_n5/RConn5
  p_n0/RConn3 -- PS-Simulink Converter39/LConn1
  p_n0/LConn1 -- p_n5/LConn1 -- p_n4/LConn1 -- p_n3/LConn1 -- p_n2/LConn1 -- Spacecraft/LConn1
  p_n0/RConn4 -- PS-Simulink Converter40/LConn1
  PS-Simulink Converter41/LConn1 -- p_n0/RConn5
  join/link 1/RConn3 -- PS-Simulink Converter23/LConn1
  joint/link2/RConn3 -- PS-Simulink Converter22/LConn1
  join/link 1/RConn4 -- PS-Simulink Converter31/LConn1
  joint/link2/RConn4 -- PS-Simulink Converter30/LConn1
  PS-Simulink Converter7/LConn1 -- joint/link2/RConn2
  join/link 1/RConn2 -- PS-Simulink Converter16/LConn1
  joint/link2/RConn1 -- p_n5/RConn1 -- joint/link3/LConn1
  Simulink-PS Converter10/RConn1 -- joint/link2/LConn2
  join/link 1/RConn1 -- joint/link2/LConn1
  join/link 1/LConn1 -- Spacecraft/RConn1
  join/link 1/LConn2 -- Simulink-PS Converter11/RConn1
  joint/link7/RConn4 -- PS-Simulink Converter24/LConn1
  joint/link7/RConn3 -- PS-Simulink Converter17/LConn1
  joint/link7/RConn2 -- PS-Simulink Converter1/LConn1
  joint/link6/LConn2 -- Simulink-PS Converter6/RConn1
  joint/link6/RConn2 -- PS-Simulink Converter2/LConn1
  joint/link6/RConn1 -- joint/link7/LConn1
  joint/link3/RConn4 -- PS-Simulink Converter29/LConn1
  joint/link3/RConn3 -- PS-Simulink Converter21/LConn1
  joint/link3/RConn2 -- PS-Simulink Converter6/LConn1
  joint/link4/RConn4 -- PS-Simulink Converter28/LConn1
  joint/link4/RConn3 -- PS-Simulink Converter20/LConn1
  joint/link4/RConn2 -- PS-Simulink Converter4/LConn1
  joint/link5/RConn4 -- PS-Simulink Converter27/LConn1
  joint/link5/RConn3 -- PS-Simulink Converter19/LConn1
  joint/link5/RConn2 -- PS-Simulink Converter3/LConn1
  joint/link6/RConn4 -- PS-Simulink Converter9/LConn1
  joint/link6/RConn3 -- PS-Simulink Converter18/LConn1
  Simulink-PS Converter7/RConn1 -- joint/link5/LConn2
  Base Sensing1/RConn6 -- PS-Simulink Converter26/LConn1
  Base Sensing1/RConn8 -- PS-Simulink Converter8/LConn1
  Base Sensing1/RConn9 -- PS-Simulink Converter11/LConn1
  Base Sensing1/RConn4 -- PS-Simulink Converter14/LConn1
  Simulink-PS Converter5/RConn1 -- joint/link7/LConn2
  Base Sensing1/RConn3 -- PS-Simulink Converter13/LConn1
  Base Sensing1/RConn11 -- PS-Simulink Converter10/LConn1
  p_n2/RConn1 -- joint/link5/RConn1 -- joint/link6/LConn1
  Base Sensing1/RConn7 -- PS-Simulink Converter5/LConn1
  Base Sensing1/RConn5 -- PS-Simulink Converter15/LConn1
  p_n3/RConn1 -- joint/link4/RConn1 -- joint/link5/LConn1
  Base Sensing1/RConn2 -- PS-Simulink Converter25/LConn1
  Simulink-PS Converter8/RConn1 -- joint/link4/LConn2
  Simulink-PS Converter9/RConn1 -- joint/link3/LConn2
  Base Sensing1/RConn10 -- PS-Simulink Converter12/LConn1
  joint/link3/RConn1 -- p_n4/RConn1 -- joint/link4/LConn1
  joint/link7/RConn1 -- Base Sensing1/RConn1 -- p_n0/RConn1
  Base Sensing1/LConn1 -- Spacecraft/LConn2 -- Conn1/RConn1

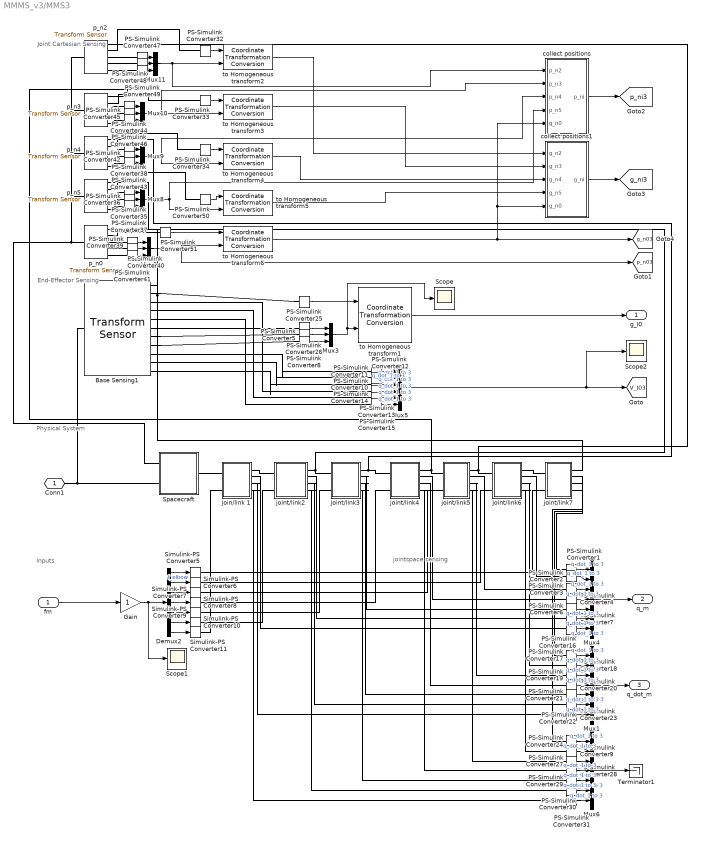
== system MMMS_v3/MMS3 ==
  note: Physical System
  note: jointspace sensing
  note: Inputs
  note: End-Effector Sensing
  note: Joint Cartesian Sensing
  fm : Inport
  Base Sensing1 : sm_lib/Frames and Transforms/Transform Sensor  MeasurementFrame=NonRotatingBase  RotationSequence=XYZ  SenseAngle=off  SenseAxis=off  SenseQ=off  SenseR=on  SenseRotationSequence=off  SenseOmegaX=on  SenseOmegaY=on  SenseOmegaZ=on  SenseOmega=off  SenseQDot=off  SenseRDot=off  SenseRotationSequenceDot=off  SenseAlphaX=off  SenseAlphaY=off  SenseAlphaZ=off  SenseAlpha=off  SenseQDDot=off  SenseRDDot=off  SenseX=on  SenseY=on  SenseZ=on  SenseXYZ=off  SenseRad=off  SenseAzim=off  SenseDist=off  SenseInc=off  SenseXDot=on  SenseYDot=on  SenseZDot=on  SenseXYZDot=off  SenseRadDot=off  SenseAzimDot=off  SenseDistDot=off  SenseIncDot=off  SenseXDDot=off  SenseYDDot=off  SenseZDDot=off  SenseXYZDDot=off  SenseRadDDot=off  SenseAzimDDot=off  SenseDistDDot=off  SenseIncDDot=off
  Demux2 : Demux  Outputs=7
  Gain : Gain
  Mux1 : Mux  Inputs=7
  Mux{2..3,8..11} (6 alike) : Mux  Inputs=3
  Mux4 : Mux  Inputs=7
  Mux5 : Mux  Inputs=6
  Mux6 : Mux  Inputs=7
  PS-Simulink Converter{1..51} (51 alike) : nesl_utility/PS-Simulink Converter  PhysicalDomain=network_engine_domain  SubClassName=ps_output  LeftPortType=input  RightPortType=output  PseudoPeriodic=off  Frequencies=[]  VectorFormat=1-D array  Unit=inherit  AffineConversion=off
  Scope : Scope
  Scope1 : Scope
  Scope2 : Scope
  Simulink-PS Converter{5..11} (7 alike) : nesl_utility/Simulink-PS Converter  PhysicalDomain=network_engine_domain  SubClassName=ps_input  LeftPortType=input  RightPortType=output  PseudoPeriodic=off  Frequencies=[]  NoiseDistribution=none  NoiseParameters=[]  Unit=1  AffineConversion=off  FilteringAndDerivatives=provide  SimscapeFilterOrder=1  InputFilterTimeConstant=0.001  UdotUserProvided=0
  Spacecraft : Subsystem
  Terminator1 : Terminator
  collect positions : MATLAB Function  TreatAsAtomicUnit=on
  collect positions1 : MATLAB Function  TreatAsAtomicUnit=on
  join/link 1 : Subsystem
  joint/link2 : Subsystem
  joint/link3 : Subsystem
  joint/link4 : Subsystem
  joint/link5 : Subsystem
  joint/link6 : Subsystem
  joint/link7 : Subsystem
  p_n{0,2..5} (5 alike) : sm_lib/Frames and Transforms/Transform Sensor  MeasurementFrame=Base  RotationSequence=XYZ  SenseAngle=off  SenseAxis=off  SenseQ=off  SenseR=on  SenseRotationSequence=off  SenseOmegaX=off  SenseOmegaY=off  SenseOmegaZ=off  SenseOmega=off  SenseQDot=off  SenseRDot=off  SenseRotationSequenceDot=off  SenseAlphaX=off  SenseAlphaY=off  SenseAlphaZ=off  SenseAlpha=off  SenseQDDot=off  SenseRDDot=off  SenseX=on  SenseY=on  SenseZ=on  SenseXYZ=off  SenseRad=off  SenseAzim=off  SenseDist=off  SenseInc=off  SenseXDot=off  SenseYDot=off  SenseZDot=off  SenseXYZDot=off  SenseRadDot=off  SenseAzimDot=off  SenseDistDot=off  SenseIncDot=off  SenseXDDot=off  SenseYDDot=off  SenseZDDot=off  SenseXYZDDot=off  SenseRadDDot=off  SenseAzimDDot=off  SenseDistDDot=off  SenseIncDDot=off
  to Homogeneous transform{1..6} (6 alike) : robotcorelib/Coordinate Transformation Conversion  InputRepresentation=Rotation Matrix  InputEulerSequence=ZYX  ShowTrVecInputPort=on  OutputRepresentation=Homogeneous Transformation  OutputEulerSequence=ZYX  ShowTrVecOutputPort=on  SimulateUsing=Code generation
  Conn1 : PMIOPort  Side=Left
  g_I0 : Outport
  q_m : Outport  Port=2
  q_dot_m : Outport  Port=3
  tag scope: V_I03=global, g_n03=global, g_ni3=global, p_n03=global, p_ni3=global
  wires:
  Demux2/1 -> Simulink-PS Converter5/1
  Demux2/3 -> Simulink-PS Converter7/1
  PS-Simulink Converter15/1 -> Mux5/6  "q_dot_1 to 3"
  PS-Simulink Converter10/1 -> Mux5/3  "q_dot_1 to 3"
  fm/1 -> Gain/1
  PS-Simulink Converter25/1 -> to Homogeneous transform1/1
  Gain/1 -> Scope1/1, Demux2/1
  PS-Simulink Converter8/1 -> Mux3/3
  Mux3/1 -> Scope/1, to Homogeneous transform1/2
  PS-Simulink Converter12/1 -> Mux5/2  "q_dot_1 to 3"
  to Homogeneous transform1/1 -> g_I0/1
  PS-Simulink Converter13/1 -> Mux5/4  "q_dot_1 to 3"
  PS-Simulink Converter26/1 -> Mux3/1
  Demux2/7 -> Simulink-PS Converter11/1
  PS-Simulink Converter14/1 -> Mux5/5  "q_dot_1 to 3"
  Demux2/4 -> Simulink-PS Converter8/1
  PS-Simulink Converter11/1 -> Mux5/1  "q_dot_1 to 3"
  PS-Simulink Converter5/1 -> Mux3/2
  Demux2/6 -> Simulink-PS Converter10/1
  Demux2/2 -> Simulink-PS Converter6/1  "f_elbow"
  Demux2/5 -> Simulink-PS Converter9/1
  PS-Simulink Converter27/1 -> Mux6/3  "q_dot_1 to 3"
  PS-Simulink Converter1/1 -> Mux4/1  "q_dot_1 to 3"
  PS-Simulink Converter6/1 -> Mux4/5  "q_dot_1 to 3"
  PS-Simulink Converter30/1 -> Mux6/6  "q_dot_1 to 3"
  PS-Simulink Converter3/1 -> Mux4/3  "q_dot_1 to 3"
  PS-Simulink Converter18/1 -> Mux1/2  "q_dot_1 to 3"
  PS-Simulink Converter31/1 -> Mux6/7  "q_dot_1 to 3"
  PS-Simulink Converter9/1 -> Mux6/2  "q_dot_1 to 3"
  PS-Simulink Converter7/1 -> Mux4/6  "q_dot_1 to 3"
  PS-Simulink Converter2/1 -> Mux4/2  "q_dot_1 to 3"
  PS-Simulink Converter4/1 -> Mux4/4  "q_dot_1 to 3"
  PS-Simulink Converter21/1 -> Mux1/5  "q_dot_1 to 3"
  PS-Simulink Converter23/1 -> Mux1/7  "q_dot_1 to 3"
  PS-Simulink Converter16/1 -> Mux4/7  "q_dot_1 to 3"
  PS-Simulink Converter28/1 -> Mux6/4  "q_dot_1 to 3"
  Mux4/1 -> q_m/1
  Mux1/1 -> q_dot_m/1
  PS-Simulink Converter24/1 -> Mux6/1  "q_dot_1 to 3"
  Mux6/1 -> Terminator1/1
  PS-Simulink Converter20/1 -> Mux1/4  "q_dot_1 to 3"
  PS-Simulink Converter29/1 -> Mux6/5  "q_dot_1 to 3"
  PS-Simulink Converter22/1 -> Mux1/6  "q_dot_1 to 3"
  PS-Simulink Converter17/1 -> Mux1/1  "q_dot_1 to 3"
  PS-Simulink Converter19/1 -> Mux1/3  "q_dot_1 to 3"
  Mux5/1 -> [V_I03], Scope2/1
  Mux2/1 -> to Homogeneous transform6/2, [p_n03]
  PS-Simulink Converter39/1 -> Mux2/1
  PS-Simulink Converter40/1 -> Mux2/2
  PS-Simulink Converter41/1 -> Mux2/3
  PS-Simulink Converter36/1 -> Mux8/2
  PS-Simulink Converter35/1 -> Mux8/1
  PS-Simulink Converter37/1 -> Mux8/3
  PS-Simulink Converter42/1 -> Mux9/2
  PS-Simulink Converter38/1 -> Mux9/1
  PS-Simulink Converter43/1 -> Mux9/3
  PS-Simulink Converter45/1 -> Mux10/2
  PS-Simulink Converter44/1 -> Mux10/1
  PS-Simulink Converter46/1 -> Mux10/3
  Mux11/1 -> to Homogeneous transform2/2, collect positions/1(p_n2)
  PS-Simulink Converter48/1 -> Mux11/2
  PS-Simulink Converter47/1 -> Mux11/1
  PS-Simulink Converter49/1 -> Mux11/3
  collect positions/1(p_ni) -> [p_ni3]
  PS-Simulink Converter32/1 -> to Homogeneous transform2/1
  PS-Simulink Converter33/1 -> to Homogeneous transform3/1
  Mux10/1 -> to Homogeneous transform3/2, collect positions/2(p_n3)
  Mux9/1 -> to Homogeneous transform4/2, collect positions/3(p_n4)
  PS-Simulink Converter34/1 -> to Homogeneous transform4/1
  PS-Simulink Converter50/1 -> to Homogeneous transform5/1
  Mux8/1 -> to Homogeneous transform5/2, collect positions/4(p_n5)
  collect positions1/1(g_ni) -> [g_ni3]
  PS-Simulink Converter51/1 -> to Homogeneous transform6/1
  to Homogeneous transform6/1 -> collect positions/5(g_n0), collect positions1/5(g_n0), [g_n03]
  to Homogeneous transform2/1 -> collect positions1/1(g_n2)
  to Homogeneous transform3/1 -> collect positions1/2(g_n3)
  to Homogeneous transform4/1 -> collect positions1/3(g_n4)
  to Homogeneous transform5/1 -> collect positions1/4(g_n5)
  connections:
  Conn1/RConn1 -- Spacecraft/LConn2 -- Base Sensing1/LConn1
  p_n0/RConn1 -- Base Sensing1/RConn1 -- joint/link7/RConn1
  joint/link4/LConn1 -- p_n4/RConn1 -- joint/link3/RConn1
  Base Sensing1/RConn10 -- PS-Simulink Converter12/LConn1
  Simulink-PS Converter9/RConn1 -- joint/link3/LConn2
  Simulink-PS Converter8/RConn1 -- joint/link4/LConn2
  Base Sensing1/RConn2 -- PS-Simulink Converter25/LConn1
  joint/link5/LConn1 -- joint/link4/RConn1 -- p_n3/RConn1
  Base Sensing1/RConn5 -- PS-Simulink Converter15/LConn1
  Base Sensing1/RConn7 -- PS-Simulink Converter5/LConn1
  joint/link6/LConn1 -- joint/link5/RConn1 -- p_n2/RConn1
  Base Sensing1/RConn11 -- PS-Simulink Converter10/LConn1
  Base Sensing1/RConn3 -- PS-Simulink Converter13/LConn1
  Simulink-PS Converter5/RConn1 -- joint/link7/LConn2
  Base Sensing1/RConn4 -- PS-Simulink Converter14/LConn1
  Base Sensing1/RConn9 -- PS-Simulink Converter11/LConn1
  Base Sensing1/RConn8 -- PS-Simulink Converter8/LConn1
  Base Sensing1/RConn6 -- PS-Simulink Converter26/LConn1
  Simulink-PS Converter7/RConn1 -- joint/link5/LConn2
  joint/link6/RConn3 -- PS-Simulink Converter18/LConn1
  joint/link6/RConn4 -- PS-Simulink Converter9/LConn1
  joint/link5/RConn2 -- PS-Simulink Converter3/LConn1
  joint/link5/RConn3 -- PS-Simulink Converter19/LConn1
  joint/link5/RConn4 -- PS-Simulink Converter27/LConn1
  joint/link4/RConn2 -- PS-Simulink Converter4/LConn1
  joint/link4/RConn3 -- PS-Simulink Converter20/LConn1
  joint/link4/RConn4 -- PS-Simulink Converter28/LConn1
  joint/link3/RConn2 -- PS-Simulink Converter6/LConn1
  joint/link3/RConn3 -- PS-Simulink Converter21/LConn1
  joint/link3/RConn4 -- PS-Simulink Converter29/LConn1
  joint/link6/RConn1 -- joint/link7/LConn1
  joint/link6/RConn2 -- PS-Simulink Converter2/LConn1
  joint/link6/LConn2 -- Simulink-PS Converter6/RConn1
  joint/link7/RConn2 -- PS-Simulink Converter1/LConn1
  joint/link7/RConn3 -- PS-Simulink Converter17/LConn1
  joint/link7/RConn4 -- PS-Simulink Converter24/LConn1
  join/link 1/LConn2 -- Simulink-PS Converter11/RConn1
  join/link 1/LConn1 -- Spacecraft/RConn1
  join/link 1/RConn1 -- joint/link2/LConn1
  Simulink-PS Converter10/RConn1 -- joint/link2/LConn2
  joint/link3/LConn1 -- p_n5/RConn1 -- joint/link2/RConn1
  join/link 1/RConn2 -- PS-Simulink Converter16/LConn1
  PS-Simulink Converter7/LConn1 -- joint/link2/RConn2
  joint/link2/RConn4 -- PS-Simulink Converter30/LConn1
  join/link 1/RConn4 -- PS-Simulink Converter31/LConn1
  joint/link2/RConn3 -- PS-Simulink Converter22/LConn1
  join/link 1/RConn3 -- PS-Simulink Converter23/LConn1
  PS-Simulink Converter41/LConn1 -- p_n0/RConn5
  p_n0/RConn4 -- PS-Simulink Converter40/LConn1
  Spacecraft/LConn1 -- p_n2/LConn1 -- p_n3/LConn1 -- p_n4/LConn1 -- p_n5/LConn1 -- p_n0/LConn1
  p_n0/RConn3 -- PS-Simulink Converter39/LConn1
  PS-Simulink Converter37/LConn1 -- p_n5/RConn5
  p_n5/RConn3 -- PS-Simulink Converter35/LConn1
  p_n5/RConn4 -- PS-Simulink Converter36/LConn1
  PS-Simulink Converter43/LConn1 -- p_n4/RConn5
  p_n4/RConn3 -- PS-Simulink Converter38/LConn1
  p_n4/RConn4 -- PS-Simulink Converter42/LConn1
  PS-Simulink Converter46/LConn1 -- p_n3/RConn5
  p_n3/RConn3 -- PS-Simulink Converter44/LConn1
  p_n3/RConn4 -- PS-Simulink Converter45/LConn1
  PS-Simulink Converter49/LConn1 -- p_n2/RConn5
  p_n2/RConn3 -- PS-Simulink Converter47/LConn1
  p_n2/RConn4 -- PS-Simulink Converter48/LConn1
  PS-Simulink Converter32/LConn1 -- p_n2/RConn2
  p_n3/RConn2 -- PS-Simulink Converter33/LConn1
  p_n4/RConn2 -- PS-Simulink Converter34/LConn1
  p_n5/RConn2 -- PS-Simulink Converter50/LConn1
  p_n0/RConn2 -- PS-Simulink Converter51/LConn1
